simulink model "TS1+TS2_Stateflow_Edge_detector_mit_testparametern"  (R2012b)
settings: Solver=FixedStepDiscrete  StartTime=0.0  StopTime=5000  RelTol=1e-3
libraries: c2833xlib x2, c280xlib x2, idelinklib_tgtpref x1
settings Model: Creator=Nikolay  LastModifiedBy=Nikolay
settings DataIOCC: SaveOutput=off  SaveTime=off
settings OptimizationCC: OptimizeModelRefInitCode=on  LifeSpan=1
settings HardwareCC: ProdBitPerChar=16  ProdBitPerInt=16  ProdBitPerPointer=16  ProdLargestAtomicInteger=Integer  ProdIntDivRoundTo=Zero  ProdEndianess=LittleEndian  ProdWordSize=16  ProdHWDeviceType=Texas Instruments->C2000
settings RTWCC: SystemTargetFile=idelink_ert.tlc  GenerateMakefile=off  TemplateMakefile=none  Description=IDE Link ERT  ProcessScript=idelink_ert_make_rtw_hook
settings CodeAppCC: IgnoreCustomStorageClasses=off

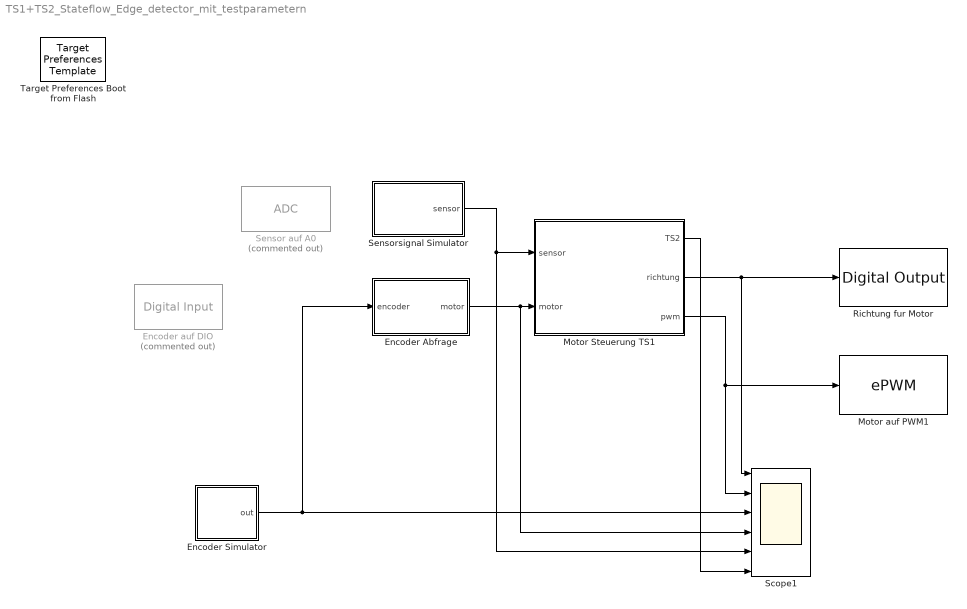
== system TS1+TS2_Stateflow_Edge_detector_mit_testparametern ==
  Encoder Abfrage : Stateflow chart  TreatAsAtomicUnit=on
  Encoder Simulator : Stateflow chart  TreatAsAtomicUnit=on
  Encoder auf DIO : c2833xlib/Digital Input  Commented=on  GPIO_Number=GPIO24~GPIO31  GPIO_Bit0=on  GPIO_Bit1=off  GPIO_Bit2=off  GPIO_Bit3=off  GPIO_Bit4=off  GPIO_Bit5=off  GPIO_Bit6=off  GPIO_Bit7=off  sampleTime=0.00001  dataType=auto  GPIO_Bit0_Qualification=Sync to SYSCLKOUT  GPIO_Bit1_Qualification=Sync to SYSCLKOUT  GPIO_Bit2_Qualification=Sync to SYSCLKOUT  GPIO_Bit3_Qualification=Sync to SYSCLKOUT  GPIO_Bit4_Qualification=Sync to SYSCLKOUT  GPIO_Bit5_Qualification=Sync to SYSCLKOUT  GPIO_Bit6_Qualification=Sync to SYSCLKOUT  GPIO_Bit7_Qualification=Sync to SYSCLKOUT  Qualification_Period=-1
  Motor Steuerung TS1 : Stateflow chart  TreatAsAtomicUnit=on
  Motor auf PWM1 : c280xlib/ePWM  checkMode=off  useModule=ePWM2  periodUnits=Clock cycles  timerSource=Specify via dialog  timerPeriod_clk=64000  timerPeriod_sec=0.0001  countingMode=Up  synchronizationOption=Disable  synchronizationEnable=off  phaseActiveEnable=Disable  phaseDirection=Count down after sync  phaseActive=0  clockPrescale=1  HSclockPrescale=1  ePWMxAStatus=on  CMPAUnits=Clock cycles  CMPASource=Specify via dialog  CMPAValue_per=50  CMPAValue_clk=32000  ePWMxAactionLogic1=Do nothing  ePWMxAactionLogic2=Clear  ePWMxAactionLogic3=Set  ePWMxAactionLogic4=Do nothing  ePWMxAactionLogic5=Do nothing  ePWMxAactionLogic6=Do nothing  ePWMxALoadMode=Load on CTR=Zero  ePWMxACSFenable=off  ePWMxACSFvalue=Forcing Disable  ePWMxASFreload=Zero  enHRPWM=off  HRPWM_LoadMode=CTR=ZERO  HRPWM_CTLMode=Phase control mode  HRPWM_EDGMode=Both edge  enSFO=on  ePWMxBStatus=on  CMPBUnits=Percentages  CMPBSource=Input port  CMPBValue_per=0  CMPBValue_clk=0  ePWMxBactionLogic1=Do nothing  ePWMxBactionLogic2=Set  ePWMxBactionLogic3=Do nothing  ePWMxBactionLogic4=Do nothing  ePWMxBactionLogic5=Clear  ePWMxBactionLogic6=Do nothing  ePWMxBLoadMode=Load on CTR=Zero  ePWMxBCSFenable=off  ePWMxBCSFvalue=Forcing Disable  ePWMxBSFreload=Zero  enableDBePWMxA=off  enableDBePWMxB=off  DBpolarity=AH  DBedgeDelay=Positive  DBSource_ePWMxA=ePWMxA  DBSource_ePWMxB=ePWMxA  DBperiodSource=Specify via dialog  REDperiod=0  FEDperiod=0  adcstartModuleA=off  adcrequestEventA=First event  adcstartEventA=CTR=Zero  adcstartModuleB=off  adcrequestEventB=First event  adcstartEventB=CTR=Zero  intEn=off  intPrd=First event  intSel=CTR=Zero  chopperEnable=off  chopperFrequency=1  chopperFirstwidth=1  chopperDuty=12.5%  tripZonesource=Specify via dialog  tzselOSHT1=off  tzselOSHT2=off  tzselOSHT3=off  tzselOSHT4=off  tzselOSHT5=off  tzselOSHT6=off  tzselCBC1=off  tzselCBC2=off  tzselCBC3=off  tzselCBC4=off  tzselCBC5=off  tzselCBC6=off  enTzOstIntr=off  enTzCbcIntr=off  ePWMxAforced=No action  ePWMxBforced=No action  timerPeriod=-1  ePWMxAValue=0  ePWMxBValue=0  tripZoneoption=OSHT
  Richtung fur Motor : c2833xlib/Digital Output  GPIO_Number=GPIO16~GPIO23  GPIO_Bit0=off  GPIO_BIT0_Toggle=off  GPIO_Bit1=off  GPIO_BIT1_Toggle=off  GPIO_Bit2=off  GPIO_BIT2_Toggle=off  GPIO_Bit3=off  GPIO_BIT3_Toggle=off  GPIO_Bit4=off  GPIO_BIT4_Toggle=off  GPIO_Bit5=on  GPIO_BIT5_Toggle=off  GPIO_Bit6=off  GPIO_BIT6_Toggle=off  GPIO_Bit7=off  GPIO_BIT7_Toggle=off
  Scope1 : Scope  NumInputPorts=6
      settings: ShowLegends=on  YMin=-5~60~7.6~-5~-5~-5  YMax=5~100~8.4~5~5~5
  Sensor auf A0 : c280xlib/ADC  Commented=on  useModule=A  useMode=Sequential  sourceSOC=Software  sourceSOC1=Software  sourceSOC2=ePWMxB  xint2_ADCSOC=31  Ts=0.001  dType=uint16  postInterrupt=off  numConversionsSingle=3  numConversionsDouble=1  conv0=ADCINA0  conv1=ADCINA1  conv2=ADCINA2  conv3=ADCINA3  conv4=ADCINA4  conv5=ADCINA5  conv6=ADCINA6  conv7=ADCINA7  conv8=ADCINB0  conv9=ADCINB1  conv10=ADCINB2  conv11=ADCINB3  conv12=ADCINB4  conv13=ADCINB5  conv14=ADCINB6  conv15=ADCINB7  convAB0=ADCINA0 and ADCINB0  convAB1=ADCINA1 and ADCINB1  convAB2=ADCINA2 and ADCINB2  convAB3=ADCINA3 and ADCINB3  convAB4=ADCINA4 and ADCINB4  convAB5=ADCINA5 and ADCINB5  convAB6=ADCINA6 and ADCINB6  convAB7=ADCINA7 and ADCINB7  convA0=ADCINA0  convA1=ADCINA1  convA2=ADCINA2  convA3=ADCINA3  convA4=ADCINA4  convA5=ADCINA5  convA6=ADCINA6  convA7=ADCINA7  convB0=ADCINB0  convB1=ADCINB1  convB2=ADCINB2  convB3=ADCINB3  convB4=ADCINB4  convB5=ADCINB5  convB6=ADCINB6  convB7=ADCINB7  c28xmultiPort=off  endma=off  chdma=1
  Sensorsignal Simulator : Stateflow chart  TreatAsAtomicUnit=on
  Target Preferences Boot from Flash : idelinklib_tgtpref/Target Preferences Template  Tag=ccslinktgtpref_ccsv4  library=off
  wires:
  Motor Steuerung TS1/3(pwm) -> Motor auf PWM1/1, Scope1/2
  Motor Steuerung TS1/2(richtung) -> Richtung fur Motor/1, Scope1/1
  Encoder Abfrage/1(motor) -> Motor Steuerung TS1/2(motor), Scope1/4
  Encoder Simulator/1(out) -> Encoder Abfrage/1(encoder), Scope1/3
  Motor Steuerung TS1/1(TS2) -> Scope1/6
  Sensorsignal Simulator/1(sensor) -> Motor Steuerung TS1/1(sensor), Scope1/5

== stateflow chart TS1+TS2_Stateflow_Edge_detector_mit_testparametern/Motor Steuerung TS1 ==
  note: # Richtungsvariable: 0 - nach vorne, 1 - nach hinten
      | # Motorvariable: 0 - gesperrt, 1 - funktioniert
      | # PWM Wert im Normalbetrieb muss heueristisch bestimmt werden (einfach Testen)
  state Start
    TS2 = 0
    pwm = 60;
    richtung = 0;
  state TS2_start_und_abfrage
    TS2 =1
  state Abfrage_Wurfel_eingeladen
    sensor;
  state Motor_Stop
    pwm = 0;
  state Abfrage_motor
    motor;
  state Normalbetrieb
    richtung = 0;
    pwm = 60;
  note: # Wartezeit muss auch wie PWM bestimmt werden
  state PWM_increment
    pwm =pwm+20
  note: # Wartezeit muss auch wie PWM bestimmt werden
  state Rueckfahrt
    pwm= 80;
    richtung = 1;
  (default) -> Start
  Rueckfahrt -> Start : [ after(1,sec)]
  Start -> Abfrage_Wurfel_eingeladen
  PWM_increment -> Abfrage_Wurfel_eingeladen [order 2] : [pwm != 100]
  Abfrage_Wurfel_eingeladen -> Motor_Stop [order 2] : [sensor == 1]
  Motor_Stop -> TS2_start_und_abfrage
  Abfrage_Wurfel_eingeladen -> Abfrage_motor [order 1] : [sensor == 0]
  Normalbetrieb -> Abfrage_Wurfel_eingeladen
  Abfrage_motor -> Normalbetrieb [order 2] : [motor == 1]
  Abfrage_motor -> PWM_increment [order 1] : [after(2,sec) && motor == 0]
  PWM_increment -> Rueckfahrt [order 1] : [pwm == 100]
  data: TS2 output double; sensor input; motor input; richtung output double; pwm output double

== stateflow chart TS1+TS2_Stateflow_Edge_detector_mit_testparametern/Encoder Abfrage ==
  state Start
    motor = 1;
    encoder;
  state Signal_auslesen
    encoder_old = encoder;
  state Neuer_wert
    encoder_new = encoder;
  state Motor_gesperrt
    motor = 0;
  state Motor_laufend
    motor = 1
  (default) -> Start
  Start -> Signal_auslesen
  Motor_gesperrt -> Signal_auslesen
  Motor_laufend -> Signal_auslesen
  Signal_auslesen -> Neuer_wert : [after(10,sec)]
  Neuer_wert -> Motor_laufend [order 1] : [encoder_new - encoder_old == 1 || encoder_new - encoder_old == -1]
  Neuer_wert -> Motor_gesperrt [order 2] : [encoder_new - encoder_old == 0 ]
  data: encoder input; motor output double; encoder_new local double; encoder_old local double

== stateflow chart TS1+TS2_Stateflow_Edge_detector_mit_testparametern/Encoder Simulator ==
  state Start
    out = 1
    counter = 0
  state Low
    out = 0
  state High
    out = 1
    counter = counter +1
  state Wieder_Gesperrt
    out = 1
  (default) -> Start
  Start -> High : [after(300,sec)]
  High -> Low [order 1] : [after(1,sec) && counter <= 10]
  Low -> High : [after(1,sec) && counter <= 10]
  High -> Wieder_Gesperrt [order 2] : [counter > 10]
  data: out output double; counter local double

== stateflow chart TS1+TS2_Stateflow_Edge_detector_mit_testparametern/Sensorsignal Simulator ==
  state Start
    sensor = 0
  state Sensor_an
    sensor = 1
  (default) -> Start
  Start -> Sensor_an : [after(1000,sec)]
  data: sensor output double
